simulink model "adapt_visodo05_RC"  (Simulink 7.5)
settings: Solver=FixedStepDiscrete  StartTime=0.0  StopTime=100  FixedStep=1  RelTol=1e-3
undefined symbols (not defined in the file): L, R
libraries: simulink x2, vipmorphops x1, vipsnks x1
(part 1 of 2)
CloseFcn:
  | rtwprivate ssgencode ModelCloseRequest adapt_visodo05_batch_adapt
settings Model: Creator=jfabia02  LastModifiedBy=jfabia02  SimulationMode=external  ExtModeEnableFloating=off  ExtModeArchiveFileName=model_output  ExtModeArchiveDirName=C:\RTtools\VU-RLNX\RLNX\RLNX\Simulink Models
settings DataIOCC: ExternalInput=[t,u]
settings DebuggingCC: UnderspecifiedInitializationDetection=Simplified  UnconnectedInputMsg=none  UnconnectedOutputMsg=none  UnconnectedLineMsg=none
settings RTWCC: SystemTargetFile=rlnx.tlc  GenCodeOnly=on  TemplateMakefile=rlnx_ubuntu.tmf  Description=Linux Real-Time Target  GenerateReport=on  ProcessScript=rlnx_make_rtw_hook  LaunchReport=on
settings CodeAppCC: GenerateComments=off  SimulinkBlockComments=off
settings STFCustomTargetCC: TargetFunctionLibrary=GNU99 (GNU)  ModelReferenceCompliant=off  GeneratePreprocessorConditionals=Disable all  MatFileLogging=on  SystemTargetFile=rlnx.tlc
settings GRTTargetCC: TargetFunctionLibrary=GNU99 (GNU)  ModelReferenceCompliant=off  ParMdlRefBuildCompliant=off  CompOptLevelCompliant=off  ExtMode=on  ExtModeMexArgs='10.0.0.2'
settings CustomProperty: DataType=string  Value=-lm -ldl /matlab_includes/libfreenect/build/lib/libfreenect.so.0.0.1
settings EnumStrPairs: String=PC

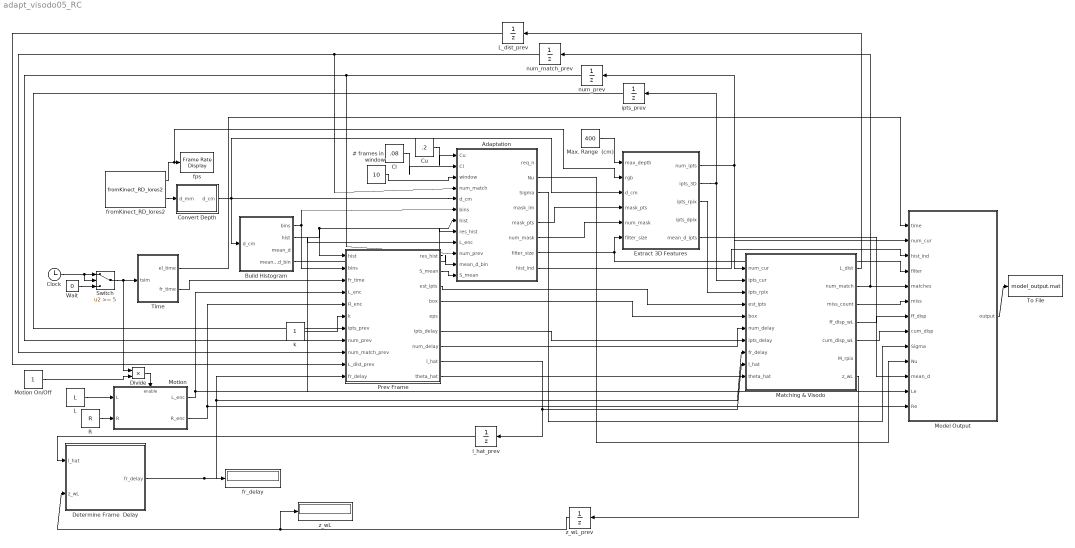
== system adapt_visodo05_RC ==
  # frames in  window : Constant  Value=10  OutDataType=fixdt(1, 16)  OutScaling=2^0
  Adaptation : Subsystem
  Build Histogram : Stateflow chart  TreatAsAtomicUnit=on
  Cl : Constant  Value=.08  OutDataType=fixdt(1, 16)  OutScaling=2^0
  Clock : Clock
      settings: Decimation=10
  Convert Depth : Subsystem
  Cu : Constant  Value=.2  OutDataType=fixdt(1, 16)  OutScaling=2^0
  Determine Frame  Delay : Stateflow chart  TreatAsAtomicUnit=on
  Divide : Product  Inputs=**  OutDataType=fixdt(1, 16)  OutScaling=2^-10
  Extract 3D Features : Subsystem
  L : Constant  Value=L  OutDataType=fixdt(1, 16)  OutScaling=2^0
  L_dist_prev : UnitDelay  X0=zeros(2,1000)  SampleTime=-1
  Matching & Visodo : Subsystem
  Max. Range  (cm) : Constant  Value=400  OutDataType=fixdt(1, 16)  OutScaling=2^0
  Model Output : Stateflow chart  TreatAsAtomicUnit=on
  Motion : Subsystem
  Motion On/Off : Constant  OutDataType=fixdt(1, 16)  OutScaling=2^0
  Prev Frame : Subsystem
  R : Constant  Value=R  OutDataType=fixdt(1, 16)  OutScaling=2^0
  Switch : Switch  Threshold=5  OutDataType=fixdt(1, 16)  OutScaling=2^0
  Time : Subsystem
  To File : ToFile  Filename=model_output.mat  MatrixName=output
  Wait : Constant  Value=0  OutDataType=fixdt(1, 16)  OutScaling=2^0
  fps : vipsnks/Frame Rate Display  DialogController=vipDDGCreate  DialogControllerArgs=DataTag0  UpdateRate=10
  fr_delay : Display
  fromKinect_RD_lores2 : S-Function  FunctionName=fromKinect_RD_lores2  EnableBusSupport=off
      mask Display: image(imread('C:\RTtools\VU-RLNX\RLNX\RLNX\Simulink Models\kinectimage.jpeg'))
  ipts_prev : UnitDelay  SampleTime=-1
  k : Constant  OutDataType=fixdt(1, 16)  OutScaling=2^0
  l_hat_prev : UnitDelay  SampleTime=-1
  num_match_prev : UnitDelay  SampleTime=-1
  num_prev : UnitDelay  SampleTime=-1
  z_wL : Display
  z_wL_prev : UnitDelay  SampleTime=-1
  wires:
  Max. Range  (cm)/1 -> Extract 3D Features/1(max_depth)
  Convert Depth/1(d_cm) -> Extract 3D Features/3(d_cm), Build Histogram/1(d_cm), Adaptation/5(d_cm)
  ipts_prev/1 -> Prev Frame/7(ipts_prev)
  num_prev/1 -> Prev Frame/8(num_prev), Adaptation/10(num_prev)
  k/1 -> Prev Frame/6(k)
  Build Histogram/2(hist) -> Prev Frame/1(hist), Adaptation/7(hist)
  # frames in  window/1 -> Adaptation/3(window)
  Matching & Visodo/2(num_match) -> num_match_prev/1, Model Output/5(matches)
  num_match_prev/1 -> Prev Frame/9(num_match_prev), Adaptation/4(num_match)
  Prev Frame/3(est_ipts) -> Matching & Visodo/4(est_ipts)
  Prev Frame/4(box) -> Matching & Visodo/5(box)
  Extract 3D Features/3(ipts_rpix) -> Matching & Visodo/3(ipts_rpix)
  Extract 3D Features/2(ipts_3D) -> Matching & Visodo/2(ipts_cur), ipts_prev/1
  Prev Frame/1(res_hist) -> Adaptation/8(res_hist)
  Adaptation/7(filter_size) -> Extract 3D Features/6(filter_size), Model Output/4(filter)
  Build Histogram/1(bins) -> Prev Frame/2(bins), Adaptation/6(bins)
  Matching & Visodo/1(" L_dist") -> L_dist_prev/1
  L_dist_prev/1 -> Prev Frame/10(L_dist_prev)
  Adaptation/5(mask_pts) -> Extract 3D Features/4(mask_pts)
  Adaptation/6(num_mask) -> Extract 3D Features/5(num_mask)
  Extract 3D Features/1(num_ipts) -> Matching & Visodo/1(num_cur), num_prev/1, Model Output/2(num_cur)
  Prev Frame/7(num_delay) -> Matching & Visodo/6(num_delay)
  Prev Frame/6(ipts_delay) -> Matching & Visodo/7(ipts_delay)
  Cu/1 -> Adaptation/1(Cu)
  Cl/1 -> Adaptation/2(Cl)
  Prev Frame/8(l_hat) -> Matching & Visodo/9(l_hat), l_hat_prev/1
  Prev Frame/9(theta_hat) -> Matching & Visodo/10(theta_hat)
  Build Histogram/4(mean_d_bin) -> Adaptation/11(mean_d_bin)
  Determine Frame  Delay/1(fr_delay) -> fr_delay/1, Prev Frame/11(fr_delay), Matching & Visodo/8(fr_delay)
  z_wL_prev/1 -> Determine Frame  Delay/2(z_wL), z_wL/1
  l_hat_prev/1 -> Determine Frame  Delay/1(l_hat)
  Matching & Visodo/7(z_wL) -> z_wL_prev/1
  Prev Frame/2(S_mean) -> Adaptation/12(S_mean)
  Clock/1 -> Switch/2, Switch/1
  Switch/1 -> Time/1(tsim), Divide/1
  Wait/1 -> Switch/3
  Motion On/Off/1 -> Divide/2
  L/1 -> Motion/1(L)
  R/1 -> Motion/2(R)
  Divide/1 -> Motion/Enable
  fromKinect_RD_lores2/2 -> Convert Depth/1(d_mm)
  fromKinect_RD_lores2/1 -> Extract 3D Features/2(rgb), fps/1
  Time/2(fr_time) -> Prev Frame/3(fr_time)
  Model Output/1(output) -> To File/1
  Time/1(el_time) -> Model Output/1(time)
  Adaptation/8(hist_ind) -> Model Output/3(hist_ind)
  Matching & Visodo/3(miss_count) -> Model Output/6(miss)
  Matching & Visodo/4(ff_disp_wL) -> Model Output/7(ff_disp)
  Matching & Visodo/5(cum_disp_wL) -> Model Output/8(cum_disp)
  Adaptation/2(Nu) -> Model Output/10(Nu)
  Adaptation/3(Sigma) -> Model Output/9(Sigma)
  Extract 3D Features/5(mean_d_ipts) -> Model Output/11(mean_d)
  Motion/1(L_enc) -> Prev Frame/4(L_enc), Adaptation/9(L_enc), Model Output/12(Le)
  Motion/2(R_enc) -> Prev Frame/5(R_enc), Model Output/13(Re)

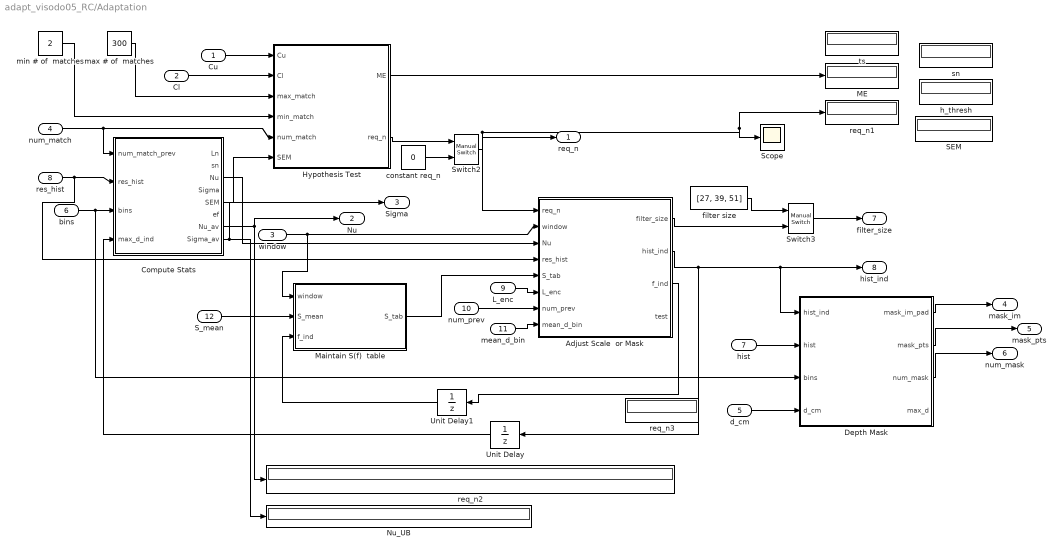
== system adapt_visodo05_RC/Adaptation ==
  Cu : Inport
  Cl : Inport  Port=2
  window : Inport  Port=3
  num_match : Inport  Port=4
  d_cm : Inport  Port=5
  bins : Inport  Port=6
  hist : Inport  Port=7  OutDataType=fixdt(1, 16)  OutScaling=2^0
  res_hist : Inport  Port=8
  L_enc : Inport  Port=9  OutDataType=fixdt(1, 16)  OutScaling=2^0
  num_prev : Inport  Port=10  OutDataType=fixdt(1, 16)  OutScaling=2^0
  mean_d_bin : Inport  Port=11  OutDataType=fixdt(1, 16)  OutScaling=2^0
  S_mean : Inport  Port=12
  Adjust Scale  or Mask : Stateflow chart  TreatAsAtomicUnit=on
  Compute Stats : Stateflow chart  TreatAsAtomicUnit=on
  Depth Mask : Stateflow chart  TreatAsAtomicUnit=on
  Hypothesis Test : Stateflow chart  TreatAsAtomicUnit=on
  ME : Display
  Maintain S(f)  table : Stateflow chart  TreatAsAtomicUnit=on
  Nu_UB : Display
  SEM : Display
  Scope : Scope
      settings: TimeRange=1000  YMin=-2  YMax=2
  Switch2 : simulink/Signal Routing/Manual Switch  SystemSampleTime=-1  sw=1  action=0  varsize=off
  Switch3 : simulink/Signal Routing/Manual Switch  SystemSampleTime=-1  sw=0  action=0  varsize=off
  Unit Delay : UnitDelay  X0=2  SampleTime=-1
  Unit Delay1 : UnitDelay  X0=2  SampleTime=-1
  constant req_n : Constant  Value=0  OutDataType=fixdt(1, 16)  OutScaling=2^0
  filter size : Constant  Value=[27, 39, 51]  VectorParams1D=off  OutDataType=fixdt(1, 16)  OutScaling=2^0
  h_thresh : Display
  max # of  matches : Constant  Value=300  OutDataType=fixdt(1, 16)  OutScaling=2^0
  min # of  matches : Constant  Value=2  OutDataType=fixdt(1, 16)  OutScaling=2^0
  req_n1 : Display
  req_n2 : Display
  req_n3 : Display
  sn : Display
  ts : Display
  req_n : Outport
  Nu : Outport  Port=2
  Sigma : Outport  Port=3
  mask_im : Outport  Port=4
  mask_pts : Outport  Port=5
  num_mask : Outport  Port=6
  filter_size : Outport  Port=7
  hist_ind : Outport  Port=8
  wires:
  Hypothesis Test/1(ME) -> ME/1
  num_match/1 -> Hypothesis Test/5(num_match), Compute Stats/1(num_match_prev)
  window/1 -> Adjust Scale  or Mask/2(window), Maintain S(f)  table/1(window)
  res_hist/1 -> Compute Stats/2(res_hist), Adjust Scale  or Mask/4(res_hist)
  bins/1 -> Compute Stats/3(bins), Depth Mask/3(bins)
  Compute Stats/3(Nu) -> Adjust Scale  or Mask/3(Nu)
  d_cm/1 -> Depth Mask/4(d_cm)
  Depth Mask/3(num_mask) -> num_mask/1
  Depth Mask/1(mask_im_pad) -> mask_im/1
  Depth Mask/2(mask_pts) -> mask_pts/1
  hist/1 -> Depth Mask/2(hist)
  Adjust Scale  or Mask/2(hist_ind) -> Unit Delay/1, hist_ind/1, Depth Mask/1(hist_ind)
  Hypothesis Test/2(req_n) -> Switch2/1
  Switch2/1 -> Adjust Scale  or Mask/1(req_n), req_n/1, Scope/1, req_n1/1
  constant req_n/1 -> Switch2/2
  Adjust Scale  or Mask/1(filter_size) -> Switch3/2
  Switch3/1 -> filter_size/1
  filter size/1 -> Switch3/1
  min # of  matches/1 -> Hypothesis Test/4(min_match)
  L_enc/1 -> Adjust Scale  or Mask/6(L_enc)
  Unit Delay/1 -> Compute Stats/4(max_d_ind)
  Compute Stats/5(SEM) -> Hypothesis Test/6(SEM)
  Cu/1 -> Hypothesis Test/1(Cu)
  num_prev/1 -> Adjust Scale  or Mask/7(num_prev)
  mean_d_bin/1 -> Adjust Scale  or Mask/8(mean_d_bin)
  Cl/1 -> Hypothesis Test/2(Cl)
  max # of  matches/1 -> Hypothesis Test/3(max_match)
  Adjust Scale  or Mask/3(f_ind) -> Unit Delay1/1
  Unit Delay1/1 -> Maintain S(f)  table/3(f_ind)
  S_mean/1 -> Maintain S(f)  table/2(S_mean)
  Maintain S(f)  table/1(S_tab) -> Adjust Scale  or Mask/5(S_tab)
  Compute Stats/7(Nu_av) -> req_n2/1, Nu/1
  Compute Stats/8(Sigma_av) -> Nu_UB/1, Sigma/1

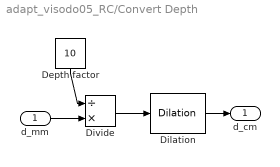
== system adapt_visodo05_RC/Convert Depth ==
  d_mm : Inport
  Depth factor : Constant  Value=10  OutDataType=fixdt(1, 16)  OutScaling=2^0
  Dilation : vipmorphops/Dilation  nhoodsrc=Specify via dialog  strel=[2 2; 2 2]
  Divide : Product  Inputs=/*  OutDataType=fixdt(1, 16)  OutScaling=2^-10
  d_cm : Outport
  wires:
  Divide/1 -> Dilation/1
  Depth factor/1 -> Divide/1
  d_mm/1 -> Divide/2
  Dilation/1 -> d_cm/1

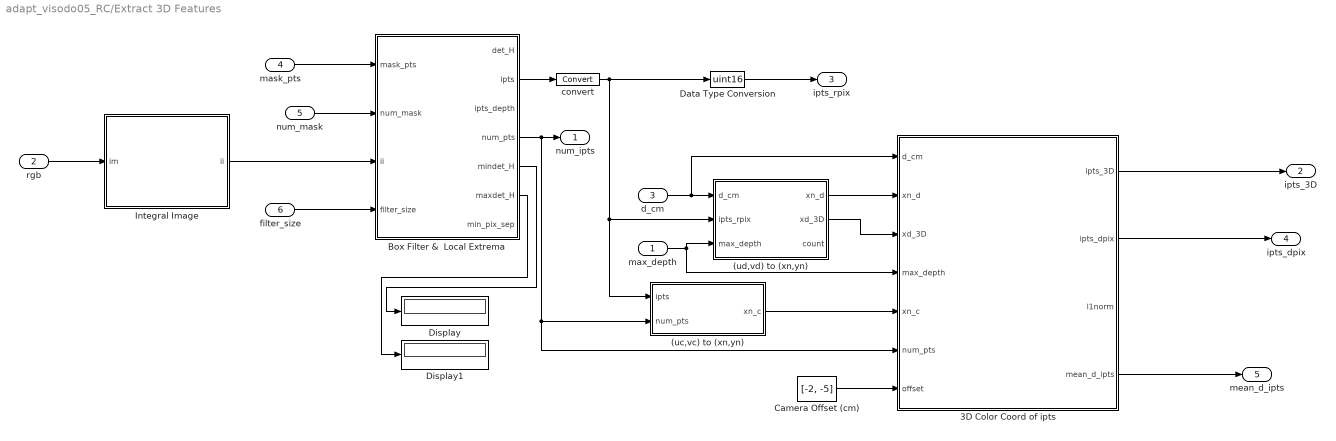
== system adapt_visodo05_RC/Extract 3D Features ==
  max_depth : Inport  OutDataType=fixdt(1, 16)  OutScaling=2^0
  rgb : Inport  Port=2
  d_cm : Inport  Port=3
  mask_pts : Inport  Port=4
  num_mask : Inport  Port=5
  filter_size : Inport  Port=6  OutDataType=fixdt(1, 16)  OutScaling=2^0
  (uc,vc) to (xn,yn) : Stateflow chart  TreatAsAtomicUnit=on
  (ud,vd) to (xn,yn) : Stateflow chart  TreatAsAtomicUnit=on
  3D Color Coord of ipts : Stateflow chart  TreatAsAtomicUnit=on
  Box Filter &  Local Extrema : Stateflow chart  TreatAsAtomicUnit=on
  Camera Offset (cm) : Constant  Value=[-2, -5]  OutDataTypeMode=double  OutDataType=fixdt(1, 16)  OutScaling=2^0  OutDataTypeStr=double
  Data Type Conversion : DataTypeConversion  OutDataTypeMode=uint16  OutDataType=fixdt(1, 16)  OutScaling=2^0  OutDataTypeStr=uint16
  Display : Display
  Display1 : Display
  Integral Image : Stateflow chart  TreatAsAtomicUnit=on
  convert : DataTypeConversion  OutDataType=fixdt(1, 16)  OutScaling=2^0
  num_ipts : Outport
  ipts_3D : Outport  Port=2
  ipts_rpix : Outport  Port=3
  ipts_dpix : Outport  Port=4
  mean_d_ipts : Outport  Port=5
  wires:
  rgb/1 -> Integral Image/1(im)
  filter_size/1 -> Box Filter &  Local Extrema/4(filter_size)
  Box Filter &  Local Extrema/2(ipts) -> convert/1
  Data Type Conversion/1 -> ipts_rpix/1
  Box Filter &  Local Extrema/4(num_pts) -> num_ipts/1, (uc,vc) to (xn,yn)/2(num_pts), 3D Color Coord of ipts/6(num_pts)
  Integral Image/1(ii) -> Box Filter &  Local Extrema/3(ii)
  mask_pts/1 -> Box Filter &  Local Extrema/1(mask_pts)
  num_mask/1 -> Box Filter &  Local Extrema/2(num_mask)
  (ud,vd) to (xn,yn)/1(xn_d) -> 3D Color Coord of ipts/2(xn_d)
  (ud,vd) to (xn,yn)/2(xd_3D) -> 3D Color Coord of ipts/3(xd_3D)
  (uc,vc) to (xn,yn)/1(xn_c) -> 3D Color Coord of ipts/5(xn_c)
  d_cm/1 -> (ud,vd) to (xn,yn)/1(d_cm), 3D Color Coord of ipts/1(d_cm)
  Camera Offset (cm)/1 -> 3D Color Coord of ipts/7(offset)
  max_depth/1 -> (ud,vd) to (xn,yn)/3(max_depth), 3D Color Coord of ipts/4(max_depth)
  3D Color Coord of ipts/1(ipts_3D) -> ipts_3D/1
  convert/1 -> Data Type Conversion/1, (ud,vd) to (xn,yn)/2(ipts_rpix), (uc,vc) to (xn,yn)/1(ipts)
  Box Filter &  Local Extrema/5(mindet_H) -> Display/1
  Box Filter &  Local Extrema/6(maxdet_H) -> Display1/1
  3D Color Coord of ipts/2(ipts_dpix) -> ipts_dpix/1
  3D Color Coord of ipts/4(mean_d_ipts) -> mean_d_ipts/1

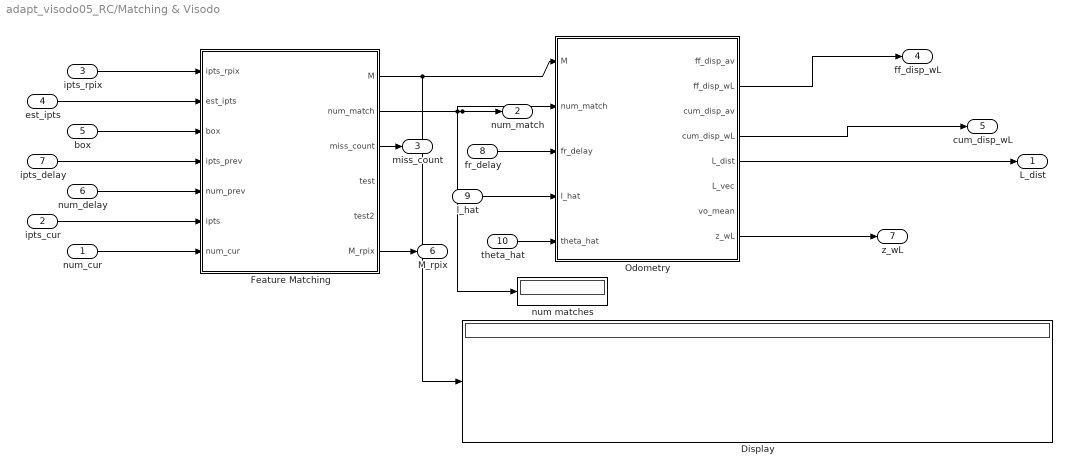
== system adapt_visodo05_RC/Matching & Visodo ==
  num_cur : Inport
  ipts_cur : Inport  Port=2
  ipts_rpix : Inport  Port=3  OutDataType=fixdt(1, 16)  OutScaling=2^0
  est_ipts : Inport  Port=4
  box : Inport  Port=5
  num_delay : Inport  Port=6
  ipts_delay : Inport  Port=7
  fr_delay : Inport  Port=8
  l_hat : Inport  Port=9
  theta_hat : Inport  Port=10
  Display : Display
  Feature Matching : Stateflow chart  TreatAsAtomicUnit=on
  Odometry : Stateflow chart  TreatAsAtomicUnit=on
  num matches : Display
  " L_dist" : Outport
  num_match : Outport  Port=2
  miss_count : Outport  Port=3
  ff_disp_wL : Outport  Port=4
  cum_disp_wL : Outport  Port=5
  M_rpix : Outport  Port=6  PortDimensions=[2 1000]
  z_wL : Outport  Port=7
  wires:
  Feature Matching/3(miss_count) -> miss_count/1
  Feature Matching/1(M) -> Odometry/1(M), Display/1
  Feature Matching/2(num_match) -> num_match/1, Odometry/2(num_match), num matches/1
  ipts_rpix/1 -> Feature Matching/1(ipts_rpix)
  ipts_cur/1 -> Feature Matching/6(ipts)
  num_cur/1 -> Feature Matching/7(num_cur)
  ipts_delay/1 -> Feature Matching/4(ipts_prev)
  num_delay/1 -> Feature Matching/5(num_prev)
  est_ipts/1 -> Feature Matching/2(est_ipts)
  box/1 -> Feature Matching/3(box)
  Odometry/5(L_dist) -> " L_dist"/1
  Feature Matching/6(M_rpix) -> M_rpix/1
  Odometry/2(ff_disp_wL) -> ff_disp_wL/1
  Odometry/4(cum_disp_wL) -> cum_disp_wL/1
  fr_delay/1 -> Odometry/3(fr_delay)
  l_hat/1 -> Odometry/4(l_hat)
  theta_hat/1 -> Odometry/5(theta_hat)
  Odometry/8(z_wL) -> z_wL/1

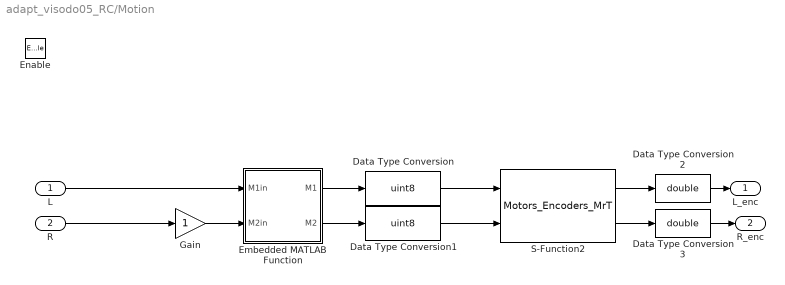
== system adapt_visodo05_RC/Motion ==
  L : Inport  OutDataType=fixdt(1, 16)  OutScaling=2^0
  R : Inport  Port=2  OutDataType=fixdt(1, 16)  OutScaling=2^0
  Enable : EnablePort
  Data Type Conversion : DataTypeConversion  OutDataTypeMode=uint8  OutDataType=fixdt(1, 16)  OutScaling=2^0  OutDataTypeStr=uint8
  Data Type Conversion1 : DataTypeConversion  OutDataTypeMode=uint8  OutDataType=fixdt(1, 16)  OutScaling=2^0  OutDataTypeStr=uint8
  Data Type Conversion2 : DataTypeConversion  OutDataTypeMode=double  OutDataType=fixdt(1, 16)  OutScaling=2^0  OutDataTypeStr=double
  Data Type Conversion3 : DataTypeConversion  OutDataTypeMode=double  OutDataType=fixdt(1, 16)  OutScaling=2^0  OutDataTypeStr=double
  Embedded MATLAB Function : Stateflow chart  TreatAsAtomicUnit=on
  Gain : Gain  ParameterDataType=fixdt(1, 16)  ParameterScaling=2^0  OutDataType=fixdt(1, 16)  OutScaling=2^0
  S-Function2 : S-Function  FunctionName=Motors_Encoders_MrT  EnableBusSupport=off
  L_enc : Outport  InitialOutput=0
  R_enc : Outport  Port=2  InitialOutput=0
  wires:
  L/1 -> Embedded MATLAB Function/1(M1in)
  Gain/1 -> Embedded MATLAB Function/2(M2in)
  Data Type Conversion1/1 -> S-Function2/2
  Data Type Conversion/1 -> S-Function2/1
  Embedded MATLAB Function/2(M2) -> Data Type Conversion1/1
  Embedded MATLAB Function/1(M1) -> Data Type Conversion/1
  S-Function2/1 -> Data Type Conversion2/1
  S-Function2/2 -> Data Type Conversion3/1
  R/1 -> Gain/1
  Data Type Conversion2/1 -> L_enc/1
  Data Type Conversion3/1 -> R_enc/1

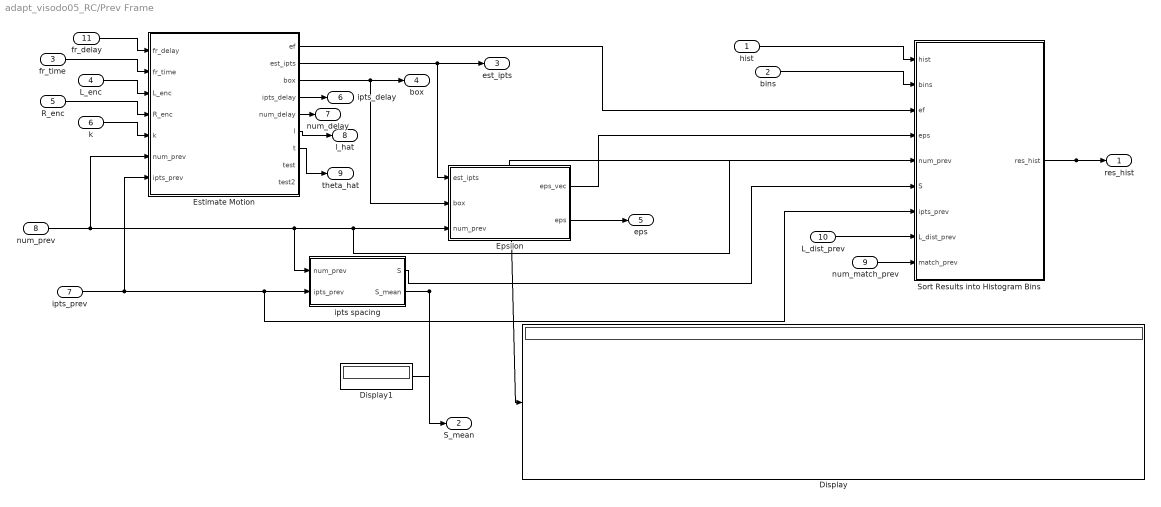
== system adapt_visodo05_RC/Prev Frame ==
  hist : Inport
  bins : Inport  Port=2
  fr_time : Inport  Port=3
  L_enc : Inport  Port=4
  R_enc : Inport  Port=5
  k : Inport  Port=6
  ipts_prev : Inport  Port=7
  num_prev : Inport  Port=8
  num_match_prev : Inport  Port=9
  L_dist_prev : Inport  Port=10
  fr_delay : Inport  Port=11
  Display : Display
  Display1 : Display
  Epsilon : Stateflow chart  TreatAsAtomicUnit=on
  Estimate Motion : Stateflow chart  TreatAsAtomicUnit=on
  Sort Results into Histogram Bins : Stateflow chart  TreatAsAtomicUnit=on
  ipts spacing : Stateflow chart  TreatAsAtomicUnit=on
  res_hist : Outport
  S_mean : Outport  Port=2
  est_ipts : Outport  Port=3
  box : Outport  Port=4
  eps : Outport  Port=5
  ipts_delay : Outport  Port=6
  num_delay : Outport  Port=7
  l_hat : Outport  Port=8
  theta_hat : Outport  Port=9
  wires:
  Estimate Motion/2(est_ipts) -> est_ipts/1, Epsilon/1(est_ipts)
  Sort Results into Histogram Bins/1(res_hist) -> res_hist/1, Display/1
  num_prev/1 -> ipts spacing/1(num_prev), Epsilon/3(num_prev), Sort Results into Histogram Bins/5(num_prev), Estimate Motion/6(num_prev)
  ipts_prev/1 -> ipts spacing/2(ipts_prev), Sort Results into Histogram Bins/7(ipts_prev), Estimate Motion/7(ipts_prev)
  hist/1 -> Sort Results into Histogram Bins/1(hist)
  Estimate Motion/1(ef) -> Sort Results into Histogram Bins/3(ef)
  ipts spacing/1(S) -> Sort Results into Histogram Bins/6(S)
  Epsilon/1(eps_vec) -> Sort Results into Histogram Bins/4(eps)
  bins/1 -> Sort Results into Histogram Bins/2(bins)
  L_dist_prev/1 -> Sort Results into Histogram Bins/8(L_dist_prev)
  num_match_prev/1 -> Sort Results into Histogram Bins/9(match_prev)
  Estimate Motion/5(num_delay) -> num_delay/1
  fr_delay/1 -> Estimate Motion/1(fr_delay)
  fr_time/1 -> Estimate Motion/2(fr_time)
  L_enc/1 -> Estimate Motion/3(L_enc)
  R_enc/1 -> Estimate Motion/4(R_enc)
  k/1 -> Estimate Motion/5(k)
  Estimate Motion/3(box) -> box/1, Epsilon/2(box)
  Estimate Motion/4(ipts_delay) -> ipts_delay/1
  Epsilon/2(eps) -> eps/1
  Estimate Motion/6(l) -> l_hat/1
  Estimate Motion/7(t) -> theta_hat/1
  ipts spacing/2(S_mean) -> Display1/1, S_mean/1

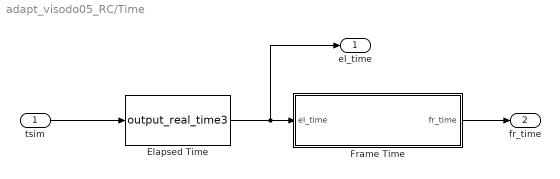
== system adapt_visodo05_RC/Time ==
  tsim : Inport  OutDataType=fixdt(1, 16)  OutScaling=2^0
  Elapsed Time : S-Function  FunctionName=output_real_time3  EnableBusSupport=off
  Frame Time : Stateflow chart  TreatAsAtomicUnit=on
  el_time : Outport
  fr_time : Outport  Port=2
  wires:
  tsim/1 -> Elapsed Time/1
  Elapsed Time/1 -> Frame Time/1(el_time), el_time/1
  Frame Time/1(fr_time) -> fr_time/1

== matlab function Build Histogram ==
  data: bins output double; d_cm input double; hist output double; mean_d output double; mean_d_bin output double
function [bins,hist, mean_d, mean_d_bin] = hist(d_cm)
% function builds histogram with non-uniform bins

% Q=1.4e-5*z^2
% 1.4e-5(z2^2 - z1^2) = C  %% constant change in Q over each bin
% if first bin is 50-125cm...
% C=0.18375  ===>  z2 = sqrt(13125+z1^2);

persistent z_pers
if isempty(z_pers)
    z_pers=zeros(2,19);
    z_pers(:,1)=[50; 125];
    for i=2:19
        z_pers(1,i)=z_pers(2,i-1); % front of bin
        z_pers(2,i)=sqrt(13125+z_pers(1,i)^2); % back of bin
    end
end
z=z_pers;

h=size(d_cm,1);
w=size(d_cm,2);
hist=zeros(1,19);
bins=zeros(2,19);
hist_pix=0;
sum_d=0;

for i=1:w
    for j=1:h
        n=1;
        if d_cm(j,i)<50 || d_cm(j,i)>500
            break
        else
            hist_pix=hist_pix+1; % counter of pixels in histogram
            sum_d=sum_d+d_cm(j,i); % running sum of depth of pixels in histogram
            for n=1:19
                z2=z(2,n);
                if d_cm(j,i)<=z2
                    hist(1,n)=hist(1,n)+1;
                    break
                end
            end
        end
    end
end
% calculate average depth of pixels in histogram and find associated bin
mean_d=sum_d/hist_pix;
mean_d_bin=1;
for n=1:19
    z2=z(2,n);
    if mean_d<=z2
        mean_d_bin=n;
        break
    end
end
bins(1:2,:)=z;

== matlab function Determine Frame Delay ==
  data: l_hat input double; fr_delay output double; z_wL input double
function fr_delay = calc_fr_delay(l_hat, z_wL)
% function calculates necessary frame delay based on weighted mean depth of matches, z_wL,
%   and estimated motion from encoders, l_hat

Qz_wL=1.4e-5*(z_wL)^2; % quantization error in depth sensor at weighted mean depth of matches

if l_hat==0
    fr_delay=0;
else
    fr_delay=ceil(Qz_wL/l_hat)+2;
end

if fr_delay>9
    fr_delay=9;
elseif isnan(fr_delay)
    fr_delay=0;
end

== matlab function Adaptation/Hypothesis Test ==
  data: Cu input double; Cl input double; max_match input double; min_match input double; ME output double; num_match input double; SEM input double; req_n output double
function [ME, req_n] = req_num(Cu,Cl,max_match,min_match,num_match,SEM)
% function determines whether or not there are a sufficient number of ipts
%   req_n=-1 ==> not enough features
%   req_n= 0 ==> number of features is just right
%   req_n= 1 ==> too many features

req_n=0;

persistent t_l
if isempty(t_l) %LUT of t_scores
    t_l=[12.71 4.303 3.182 2.776 2.571 2.447 2.365 2.306 2.262 2.228 2.201 2.179 ...
        2.16 2.145 2.131 2.12 2.11 2.101 2.093 2.086 2.08 2.074 2.069 2.064 2.06 ...
        2.056 2.052 2.048 2.045 2.042]; 
end

n=num_match;
df=n-1;

if n<=30 && n>=min_match
    ta2=t_l(df); % t_alpha/2
elseif n>30
    ta2=1.96;
else
    ta2=0;
end
ME=ta2*SEM; % margin of error

% hypothesis test
if n<min_match
    req_n=-1;
elseif n>max_match
    req_n=1;
else
    if ME>Cu % insufficient matches
        req_n=-1;
    elseif ME<=Cu && ME>=Cl % just right
        req_n=0;
    elseif ME<Cl % too many matches
        req_n=1;
    end
end

== matlab function Extract 3D Features/Integral Image ==
  data: im input double; ii output double
function ii = integral_image(im)
% function input is image, im
% output is integral image, ii
im = double(im);
height = size(im,1);
width = size(im,2);
ii = double(zeros(height, width));
col_sum = zeros(height,1);

ii(1,1) = double(im(1,1));
% first column
for j = 2:height
    ii(j,1) = im(j,1) + ii(j-1,1);
end
% first row
for i = 2:width
    ii(1,i) = im(1,i) + ii(1, i-1);
end
% rest of image
for i = 2:width
    col_sum(1,1) = im(1,i);
    for j = 2:height
        col_sum(j,1) = im(j,i) + col_sum(j-1,1);
        ii(j,i) = col_sum(j,1) + ii(j,i-1);
    end
end

== matlab function Extract 3D Features/Box Filter & Local Extrema ==
  data: mask_pts input double; num_mask input double; det_H output double; ipts output double; ipts_depth output double; ii input double; filter_size input double; num_pts output double; mindet_H output double; maxdet_H output double; min_pix_sep output double

function [det_H, ipts,ipts_depth, num_pts, mindet_H, maxdet_H, min_pix_sep]  = box_filter(mask_pts,num_mask,ii, filter_size)
% input is integral image calculated in 'Integral Image'
% ipts across 3 scales:
%   - either 15, 27, 39 
%   - or 27, 39, 51

%%%%%%%%%%%%%%%%%%%%%%%%%%%%%%%%%%%%%%%%%%%%%%%%%%%%%%%%%%%%%%%%%%%%%%%
pos_thres = 0;  % use this threshold to fire on high-contrast areas
neg_thres = 0; % det_H range is generally not symmetric about zero
max_num_ipts = 1000; %%%%% 
min_sep = 0; %% minimum separation, in pixels, between adjacent ipts
%%%%%%%%%%%%%%%%%%%%%%%%%%%%%%%%%%%%%%%%%%%%%%%%%%%%%%%%%%%%%%%%%%%%%%%


h = size(ii,1);
w = size(ii,2);
ipts = uint16(zeros(2,max_num_ipts));
ipts_depth=zeros(1,max_num_ipts);
num_pts = 0;
count = 0;
mask=mask_pts;
min_pix_sep=777;
det_H = zeros(h,w);
mindet_H = 0;
maxdet_H = 0;
Dyy = zeros(h,w);
Dxx = zeros(h,w);
Dxy = zeros(h,w);

persistent fs_pers mask_pts_pers
if isempty(fs_pers)
    fs_pers=zeros(1,3);
% %     fs_pers=filter_size';
    mask_pts_pers=zeros(2,h*w);
    c=0;
    for y=1:h
        for x=1:w
            c=c+1;
            mask_pts_pers(:,c)=[y;x];
        end
    end
end
fs_bands=zeros(2,3);
fs=[0 0 0];

% if mask is empty (off), use all points
if mask_pts(1,1)==0 && mask_pts(2,1)==0
    mask_pts=mask_pts_pers;
end

if fs_pers(1,1)==filter_size(1,1) % filter size hasn't changed
    fs_bands(1,1:3)=fs_pers(1,1:3);
    bands=1;
else
    fs_bands=[fs_pers;filter_size];
    bands=2;
end

for b=1:bands
    fs=fs_bands(b,:);
    
    det_H = zeros(h,w);
    mindet_H = 0;
    maxdet_H = 0;
    Dyy = zeros(h,w);
    Dxx = zeros(h,w);
    Dxy = zeros(h,w);    

    % calculate related filter dimensions
    fc = round(fs(2)/2);
    area = fs(2)*fs(2);
    fs2d3 = (fs(2)/3);

    fc1 = round(fs(1)/2);
    area1 = fs(1)*fs(1);
    fs1d3 = (fs(1)/3);

    fc3 = round(fs(3)/2);
    area3 = fs(3)*fs(3);
    fs3d3 = (fs(3)/3);

% % for i = fc3+1:(w-fc3)
% %     for j = fc3+1:(h-fc3)
    for m=1:num_mask
        j=mask(1,m);
        i=mask(2,m);
        if j>fc && i>fc && j<h-fc && i<w-fc
            % reference points for computing response from integral image
            % o's are Dyy pts, c's are Dxx pts, q's are Dxy pts.
            oj1 = j - fc;
            oi1 = i - (fs2d3); oi2 = oi1; oi3 = oi1; oi4 = oi1;
            oj2 = j - fc + (fs2d3);        
            oj3 = j + fc - (fs2d3)-1;        
            oj4 = j + fc - 1;        
            oj5 = oj1; oj6 = oj2; oj7 = oj3; oj8 = oj4;
            oi5 = i + (fs2d3) -1; oi6 = oi5; oi7 = oi5; oi8 = oi5;
            Dyy(j,i) = 2*(ii(oj7,oi7) - ii(oj6,oi6) -ii(oj3,oi3) + ii(oj2,oi2))...
                       - (ii(oj6,oi6) - ii(oj5,oi5) - ii(oj2,oi2) + ii(oj1,oi1))...
                       - (ii(oj8,oi8) - ii(oj7,oi7) - ii(oj4,oi4) + ii(oj3,oi3));

            ci1 = i - fc;
            cj1 = j - (fs2d3); cj2 = cj1; cj3 = cj1; cj4 = cj1;
            ci2 = i - fc + (fs2d3);        
            ci3 = i + fc - (fs2d3)-1;        
            ci4 = i + fc - 1;        
            ci5 = ci1; ci6 = ci2; ci7 = ci3; ci8 = ci4;
            cj5 = j + (fs2d3) -1; cj6 = cj5; cj7 = cj5; cj8 = cj5;
            Dxx(j,i) = 2*(ii(cj7,ci7) - ii(cj6,ci6) -ii(cj3,ci3) + ii(cj2,ci2))...
                       - (ii(cj6,ci6) - ii(cj5,ci5) - ii(cj2,ci2) + ii(cj1,ci1))...
                       - (ii(cj8,ci8) - ii(cj7,ci7) - ii(cj4,ci4) + ii(cj3,ci3));

            qi1 = i-(fs2d3)-1; qi2 = qi1; qi3 = qi1; qi4=qi1;
            qi5 = i-1; qi6=qi5; qi7=qi5; qi8=qi5;
            qi9 = i; qi10 = i; qi11=i; qi12=i;
            qi13 = i+(fs2d3); qi14=qi13; qi15=qi13; qi16=qi13;
            qj1 = j-(fs2d3)-1; qj5=qj1; qj9=qj1; qj13=qj1;
            qj2 = j-1; qj6=qj2; qj10=qj2; qj14=qj2;
            qj3=j; qj7=j; qj11=j; qj15=j;
            qj4=j+(fs2d3); qj8=qj4; qj12=qj4; qj16=qj4;
            Dxy(j,i) = (ii(qj8,qi8)-ii(qj7,qi7)-ii(qj4,qi4)+ii(qj3,qi3))...
                      + (ii(qj14,qi14)-ii(qj13,qi13)-ii(qj10,qi10)+ii(qj9,qi9))...
                      - (ii(qj6,qi6)-ii(qj5,qi5)-ii(qj2,qi2)+ii(qj1,qi1))...
                      -( ii(qj16,qi16)-ii(qj15,qi15)-ii(qj12,qi12)+ii(qj11,qi11));

            det_H(j,i) = ((Dyy(j,i) * Dxx(j,i)) - (0.81*Dxy(j,i)*Dxy(j,i)))/(area*area);
            if det_H(j,i)>maxdet_H
                maxdet_H = det_H(j,i);
            elseif det_H(j,i)<mindet_H
                mindet_H = det_H(j,i);
            end
        end % if j<....
    % % end % j
    % % end% i
    end %m
    % find local extrema 
    % % for i = fc+1:(w-fc)
    % %     for j = fc+1:(h-fc)
    for m=1:num_mask
        j=mask(1,m);
        i=mask(2,m);
        d=mask(3,m);
        if j>fc3 && i>fc3 && j<h-fc3 && i<w-fc3
            if count < max_num_ipts && i>=fc+3 && j>=fc+3 % && imd(j,i)~=0 && imd(j,i)<max_depth
                p = (det_H(j,i));
                t1 = (det_H(j-1,i-1));
                t2 = (det_H(j,i-1));
                t3 = (det_H(j+1,i-1));
                t4 = (det_H(j-1,i));
                t5 = (det_H(j+1,i));
                t6 = (det_H(j-1,i+1));
                t7 = (det_H(j,i+1));
                t8 = (det_H(j+1,i+1));

                if ((p>pos_thres && p>t1 && p>t2 && p>t3 && p>t4 ...
                   && p>t5 && p>t6 && p>t7 && p>t8) || ...
                   (p<neg_thres && p<t1 && p<t2 && p<t3 && p<t4 ...
                   && p<t5 && p<t6 && p<t7 && p<t8))% && imd(j,i)~=0 && imd(j,i)<max_depth
                    count = count +1;
                    ipts(:,count) = [j;i];
                    ipts_depth(1,count)=d;

                    % delete ipts if too close to previous ipts
                    if count>1 
                        flag=0;

                        for n=1:count-1
                            prox=abs(int16(ipts(1,n))-int16(ipts(1,count))) ...
                               + abs(int16(ipts(2,n))-int16(ipts(2,count)));
                           if prox<=min_sep && flag==0;
                                ipts(:,count) = [0;0]; 
                                ipts_depth(1,count)=0;
                                count =count-1;
                                flag=1; 
                           end
                        end
                    end
    % %             end
                % at this point, have detected ipts in middle band
                % now, need to check against bottom and top bands
                det_H1=0; Dxx1=0; Dyy1=0; Dxy1=0;
                det_H3=0; Dxx3=0; Dyy3=0; Dxy3=0;

                    % build det_H for bottom band, f=1
                    oj1 = j - fc1;
                    oi1 = i - (fs1d3); oi2 = oi1; oi3 = oi1; oi4 = oi1;
                    oj2 = j - fc1 + (fs1d3);        
                    oj3 = j + fc1 - (fs1d3)-1;        
                    oj4 = j + fc1 - 1;        
                    oj5 = oj1; oj6 = oj2; oj7 = oj3; oj8 = oj4;
                    oi5 = i + (fs1d3) -1; oi6 = oi5; oi7 = oi5; oi8 = oi5;
                    Dyy1 = 2*(ii(oj7,oi7) - ii(oj6,oi6) -ii(oj3,oi3) + ii(oj2,oi2))...
                               - (ii(oj6,oi6) - ii(oj5,oi5) - ii(oj2,oi2) + ii(oj1,oi1))...
                               - (ii(oj8,oi8) - ii(oj7,oi7) - ii(oj4,oi4) + ii(oj3,oi3));

                    ci1 = i - fc1;
                    cj1 = j - (fs1d3); cj2 = cj1; cj3 = cj1; cj4 = cj1;
                    ci2 = i - fc1 + (fs1d3);        
                    ci3 = i + fc1 - (fs1d3)-1;        
                    ci4 = i + fc1 - 1;        
                    ci5 = ci1; ci6 = ci2; ci7 = ci3; ci8 = ci4;
                    cj5 = j + (fs1d3) -1; cj6 = cj5; cj7 = cj5; cj8 = cj5;
                    Dxx1 = 2*(ii(cj7,ci7) - ii(cj6,ci6) -ii(cj3,ci3) + ii(cj2,ci2))...
                               - (ii(cj6,ci6) - ii(cj5,ci5) - ii(cj2,ci2) + ii(cj1,ci1))...
                               - (ii(cj8,ci8) - ii(cj7,ci7) - ii(cj4,ci4) + ii(cj3,ci3));

                    qi1 = i-(fs1d3)-1; qi2 = qi1; qi3 = qi1; qi4=qi1;
                    qi5 = i-1; qi6=qi5; qi7=qi5; qi8=qi5;
                    qi9 = i; qi10 = i; qi11=i; qi12=i;
                    qi13 = i+(fs1d3); qi14=qi13; qi15=qi13; qi16=qi13;
                    qj1 = j-(fs1d3)-1; qj5=qj1; qj9=qj1; qj13=qj1;
                    qj2 = j-1; qj6=qj2; qj10=qj2; qj14=qj2;
                    qj3=j; qj7=j; qj11=j; qj15=j;
                    qj4=j+(fs1d3); qj8=qj4; qj12=qj4; qj16=qj4;
                    Dxy1 = (ii(qj8,qi8)-ii(qj7,qi7)-ii(qj4,qi4)+ii(qj3,qi3))...
                              + (ii(qj14,qi14)-ii(qj13,qi13)-ii(qj10,qi10)+ii(qj9,qi9))...
                              - (ii(qj6,qi6)-ii(qj5,qi5)-ii(qj2,qi2)+ii(qj1,qi1))...
                              -( ii(qj16,qi16)-ii(qj15,qi15)-ii(qj12,qi12)+ii(qj11,qi11));

                    det_H1 = ((Dyy1 * Dxx1) - (0.81*Dxy1*Dxy1))/(area1*area1);

                    % build det_H for top band, f=3
                    oj1 = j - fc3;
                    oi1 = i - (fs3d3); oi2 = oi1; oi3 = oi1; oi4 = oi1;
                    oj2 = j - fc3 + (fs3d3);        
                    oj3 = j + fc3 - (fs3d3)-1;        
                    oj4 = j + fc3 - 1;        
                    oj5 = oj1; oj6 = oj2; oj7 = oj3; oj8 = oj4;
                    oi5 = i + (fs3d3) -1; oi6 = oi5; oi7 = oi5; oi8 = oi5;
                    Dyy3 = 2*(ii(oj7,oi7) - ii(oj6,oi6) -ii(oj3,oi3) + ii(oj2,oi2))...
                               - (ii(oj6,oi6) - ii(oj5,oi5) - ii(oj2,oi2) + ii(oj1,oi1))...
                               - (ii(oj8,oi8) - ii(oj7,oi7) - ii(oj4,oi4) + ii(oj3,oi3));

                    ci1 = i - fc3;
                    cj1 = j - (fs3d3); cj2 = cj1; cj3 = cj1; cj4 = cj1;
                    ci2 = i - fc3 + (fs3d3);        
                    ci3 = i + fc3 - (fs3d3)-1;        
                    ci4 = i + fc3 - 1;        
                    ci5 = ci1; ci6 = ci2; ci7 = ci3; ci8 = ci4;
                    cj5 = j + (fs3d3) -1; cj6 = cj5; cj7 = cj5; cj8 = cj5;
                    Dxx3 = 2*(ii(cj7,ci7) - ii(cj6,ci6) -ii(cj3,ci3) + ii(cj2,ci2))...
                               - (ii(cj6,ci6) - ii(cj5,ci5) - ii(cj2,ci2) + ii(cj1,ci1))...
                               - (ii(cj8,ci8) - ii(cj7,ci7) - ii(cj4,ci4) + ii(cj3,ci3));

                    qi1 = i-(fs3d3)-1; qi2 = qi1; qi3 = qi1; qi4=qi1;
                    qi5 = i-1; qi6=qi5; qi7=qi5; qi8=qi5;
                    qi9 = i; qi10 = i; qi11=i; qi12=i;
                    qi13 = i+(fs3d3); qi14=qi13; qi15=qi13; qi16=qi13;
                    qj1 = j-(fs3d3)-1; qj5=qj1; qj9=qj1; qj13=qj1;
                    qj2 = j-1; qj6=qj2; qj10=qj2; qj14=qj2;
                    qj3=j; qj7=j; qj11=j; qj15=j;
                    qj4=j+(fs3d3); qj8=qj4; qj12=qj4; qj16=qj4;
                    Dxy3 = (ii(qj8,qi8)-ii(qj7,qi7)-ii(qj4,qi4)+ii(qj3,qi3))...
                              + (ii(qj14,qi14)-ii(qj13,qi13)-ii(qj10,qi10)+ii(qj9,qi9))...
                              - (ii(qj6,qi6)-ii(qj5,qi5)-ii(qj2,qi2)+ii(qj1,qi1))...
                              -( ii(qj16,qi16)-ii(qj15,qi15)-ii(qj12,qi12)+ii(qj11,qi11));

                    det_H3 = ((Dyy3 * Dxx3) - (0.81*Dxy3*Dxy3))/(area3*area3);

                    % delete if ipts is not max relative to bottom and top bands
                    if (abs(p)>abs(det_H1) && abs(p)>abs(det_H3))
                        continue
                    else
                        ipts(:,count) = [0;0]; 
                        ipts_depth(1,count)=d;
                        count =count-1;      
                    end
                end
            end % if count < max_num_ipts
        end
    % %     end % i        
    % % end % j
    end % m
end %b
% compute minimum separation between adjacent pixels
for c=1:count
    for p=c+1:count
        prox=sqrt((double(ipts(1,p))-double(ipts(1,c)))^2 ...
           + (double(ipts(2,p))-double(ipts(2,c)))^2);
        
       if prox<min_pix_sep
           min_pix_sep=prox;
       end
        
    end
end

fs_pers=filter_size;
num_pts = count; % number of ipts found...could be less than max_num_ipts

== matlab function Adaptation/Maintain S(f) table ==
  data: window input double; S_mean input double; S_tab output double; f_ind input double
function S_tab = S_f_table(window, S_mean, f_ind)
% function maintains and updates table of S as function of filter scale, f

persistent S_tab_pers c_pers S_sum_pers
if isempty(S_tab_pers)
    S_tab_pers=[2 4 7 15 25 40]; % initial table of feature spacing for each scale (from empirical data)
    c_pers=0;
    S_sum_pers=0;
end

S_tab=S_tab_pers;
S_sum=S_sum_pers;;

c=c_pers; % counter inside of window
c=c+1;

if isnan(S_mean) % no features
    S_mean=0;
end

if c<window % inside of window
    S_sum=S_sum+S_mean; % running total of average spacing at current f
else % end of window
    c=0;
    S_win=S_sum/window; % average S inside of window
    S_tab(f_ind)=S_win; 
    S_sum=0;
end



S_tab_pers=S_tab;
c_pers=c;
S_sum_pers=S_sum;

== matlab function Motion/Embedded MATLAB Function ==
  data: M1in input double; M1 output double; M2in input double; M2 output double
function [M1, M2] = MotorPackets(M1in, M2in)
%#eml

M1 = 0;
M2 = 1;

if M1in>2
    M1in = 2;
elseif M1in<0
    M1in = 0;
end
if M2in>2
    M2in = 2;
elseif M2in<0
    M2in = 0;
end

gain = 2/(2^7 - 1);

M1 = M1 + round(M1in/gain)*2;
M2 = M2 + round(M2in/gain)*2;

== matlab function Extract 3D Features/(uc,vc) to (xn,yn) ==
  data: ipts input double; num_pts input double; xn_c output double size=[4 ;1000]
function xn_c  = uc_to_xn(ipts, num_pts)
% function builds LUT for xk and...
% converts ipts in (uc, vc) from 'find local extrema' into (xn, yn)


persistent xk_LUT x_inc y_inc x_init x_fin y_init y_fin uc0 vc0 fxc fyc LUT_x_steps LUT_y_steps
if isempty(xk_LUT)
    %%%% Define grid for xk_LUT %%%%%%%%
    x_inc = .01; % frame rate very sensitive to these values
    y_inc = .02;
    x_init = -0.58;
    x_fin = 0.52;
    y_init = -0.36;
    y_fin = 0.13;
    %%%%%%%%%%%%%%%%%%%%%%%%%%%%%%%%%%%%
    
    
    k1=.1925; k2=-.384; k3=.0022; k4=.0056;
    x = x_init:x_inc:x_fin;
    y = y_init:y_inc:y_fin;

    [xn, yn] = meshgrid(x,y);

    xk=xn.*(1+k1.*(xn.^2+yn.^2)+k2.*(xn.^4+yn.^4+2*xn.^2.*yn.^2)) + 2*k3.*xn.*yn + k4.*(3.*xn.^2+yn.^2);
    yk=yn.*(1+k1.*(xn.^2+yn.^2)+k2.*(xn.^4+yn.^4+2*xn.^2.*yn.^2)) + 2*k4.*xn.*yn + k3.*(3.*yn.^2+xn.^2);

    xk_LUT = zeros(size(xk,1),size(xk,2),2);
    xk_LUT(:,:,1) = xk;
    xk_LUT(:,:,2) = yk;
    
    % rgb intrinsics
    uc0 = 318.2174; vc0 = 262.5753;
    fxc = 531.5340; fyc = 529.7583;
    
    LUT_x_steps = (x_fin-x_init)/x_inc +1;
    LUT_y_steps = (y_fin-y_init)/y_inc +1;
end
max_num_ipts = 1000; %%%%% must be same for 'find_local_extrema', 'uc_to_xk' and 'ipts_to_3Dcolor'
num = max_num_ipts;

xk = zeros(1, num);
yk = zeros(1,num);
xn_c = zeros(4, num);

% convert ipts from (uc, vc) to (xk, yk)
for n = 1:num_pts

    xk(n) = (((2*double(ipts(2,n))) - uc0)/fxc); % image is 1/2 width
    yk(n) = ((2*double(ipts(1,n)+40)) - vc0)/fyc; % image is 1/2 height and cropped at row 40

% use LUT to convert (xk, yk) to (xn, yn)
    metricx = abs(xk_LUT(1,1,1)-xk(n));
    metricy = abs(xk_LUT(1,1,2)-yk(n));
    inx=1; jny=1;
    for i = 1:LUT_x_steps
        for j = 1:LUT_y_steps
            if abs(xk_LUT(j,i,1)-xk(n)) < metricx
                metricx = abs(xk_LUT(j,i,1)-xk(n));
                inx = i; % (xn, yn) indices from xk_LUT
            end
            if abs(xk_LUT(j,i,2)-yk(n)) < metricy
                metricy = abs(xk_LUT(j,i,2)-yk(n));
                jny = j; % (xn, yn) indicies from yk_LUT
            end
        end
    end
    % convert indices to metric
    xnx = x_init + (inx-1)*x_inc;
    yny = y_init + (jny-1)*y_inc;  
    % average values from xk_LUT and yk_LUT
    xn_c(:,n) = [(xnx); (yny); double(ipts(1,n)); double(ipts(2,n))];
      
end

== matlab function Extract 3D Features/(ud,vd) to (xn,yn) ==
  data: d_cm input double; ipts_rpix input double; xn_d output double; xd_3D output double; max_depth input double; count output double
function [xn_d, xd_3D, count]  = d_to_xn(d_cm, ipts_rpix, max_depth)
% function converts all points in depth image into normalized color space (xn,yn)

% define persistent variables
persistent r11 r12 r13 r21 r22 r23 r33 t1 t2 ud0 vd0 fxd fyd
if isempty(r11)
    
    % Rrel from fabian_test_results_good.mat
    r11=0.9999; r12=-0.0071; r13=-0.0078;
    r21=0.0069; r22=0.9997; r23=-0.0240;
    r33= 0.9997; %%r31=0.0080; r32=0.0239;

    % Trel from fabian_test_results_good.mat
    t1=-2.08; t2=0.04; %%t3=0.06;

    % Depth camera intrinsics
    ud0 = 324.1963; vd0 = 232.6185;
    fxd = 590.4609; fyd = 582.7801;
end
%%%%%%%%%%%%%%%%%%%%%%%
max_num_ipts = 1000;

% define ROI to search around each ipts
ROI = 10; % will create search area of (ROI+ROI+1)^2
%%%%%%%%%%%%%%%%%%%%%%%

array_size = (ROI+ROI+1)*(ROI+ROI+1);
xd_3D = zeros(array_size,max_num_ipts,3); % depth signal converted to 3D DEPTH coordinates
xn_d = zeros(array_size,max_num_ipts,2); % depth signal converted to NORMALIZED 3D COLOR coordinates

num_ipts = size(ipts_rpix,2);


count = zeros(1,max_num_ipts);
for n = 1:num_ipts
    % shorten variable names for convenience
    i_j = double(ipts_rpix(1,n));
    i_i = double(ipts_rpix(2,n));
    x=0; y=0; z=0;
    
    if i_i~=0 && i_j~=0
    for i = i_i-ROI:i_i+ROI
        for j = i_j-ROI:i_j+ROI
            count(n) = count(n) +1;
            if d_cm(j,i) <= max_depth && d_cm(j,i) ~=28483 % skip points too far away or out of range (28483)
                
                z = double(d_cm(j,i));
                x = double((z/fxd)*(i*2 - ud0));
                y = double((z/fyd)*((j+40)*2 - vd0));
                xd_3D(count(n),n,1) = x; 
                xd_3D(count(n),n,2) = y; 
                xd_3D(count(n),n,3) = z;

                D = r33*z; % approximation based on relative size of terms in D
                xn_d(count(n),n,1) = (r11*x+r12*y+r13*z+t1)/D;
                xn_d(count(n),n,2) = (r21*x+r22*y+r23*z+t2)/D;

            end
        end
    end
    end
end

== matlab function Extract 3D Features/3D Color Coord of ipts ==
  data: d_cm input double; xn_d input double; xd_3D input double; max_depth input double; xn_c input double size=[4;1000]; num_pts input double; ipts_3D output double; ipts_dpix output double size=[2 1000]; l1norm output double; offset input double; mean_d_ipts output double
function [ipts_3D, ipts_dpix, l1norm, mean_d_ipts]  = ipts_to_3Ddepth(d_cm, xn_d,xd_3D, max_depth, xn_c, num_pts, offset)
% function finds best match between ipts/xn from rgb and xn_d
% and generates 3D_DEPTH coordinates for each ipts


persistent ud0 vd0 fxd fyd
if isempty(ud0)
    % Depth camera intrinsics ('fabian_test_results_good.mat')
    ud0 = 324.1963; vd0 = 232.6185;
    fxd = 590.4609; fyd = 582.7801;
end

max_num_ipts = 1000; %%%%% must be same for 'find_local_extrema', 'uc_to_xk' and 'ipts_to_3Dcolor'
dist_thres = 20; % threshold in pixels for match between ipts_rpix and ipts_dix
ROI = 10;
x_offset=offset(1);
z_offset=offset(2);
  
array_size = (ROI+ROI+1)*(ROI+ROI+1);

ipts_3D = zeros(3,max_num_ipts);
ipts_rpix=uint16(zeros(2,max_num_ipts));
ipts_rpix = uint16(xn_c(3:4,1:max_num_ipts));
ipts_dpix = uint16(zeros(2, max_num_ipts));
l1norm = 1;

% calculate L1norm between each pair of points in xn_d and xn_c
for i = 1:num_pts % loop over all ipts
    % get pix coord of current ipts
    xnx = xn_c(1,i);
    yny = xn_c(2,i);
    i_j = xn_c(3,i);
    i_i = xn_c(4,i);
    
    l1norm = (abs(xn_d(1,i,1)-xnx) + abs(xn_d(1,i,2)-yny));

    for c = 2:array_size
            if (abs(xn_d(c,i,1)-xnx) + abs(xn_d(c,i,2)-yny)) < l1norm 
                l1norm = (abs(xn_d(c,i,1)-xnx) + abs(xn_d(c,i,2)-yny)); 
                ipts_3D(:,i) = [xd_3D(c,i,1)+x_offset; xd_3D(c,i,2); xd_3D(c,i,3)+z_offset]; % adjust for offset of camera
                ipts_dpix(1,i) = uint16((((fyd*ipts_3D(2,i)/ipts_3D(3,i)) + vd0)/2)-40);
                ipts_dpix(2,i) = uint16((fxd*(ipts_3D(1,i)/ipts_3D(3,i)) + ud0)/2);
            end
    end
        
    % zero out bad matches
% %     if (abs(ipts_dpix(1,i)-i_j) + abs(ipts_dpix(2,i)-i_i)) > (dist_thres) ...
% %        || d_cm(ipts_dpix(1,i),ipts_dpix(2,i))>=max_depth
% %         ipts_dpix(:,i) = [0;0];
% %         ipts_rpix(:,i) = [0;0];
% %         ipts_3D(:,i) = [0;0;0];
% %     end
end

mean_d_ipts=mean(ipts_3D(3,1:num_pts));

== matlab function Prev Frame/Estimate Motion ==
  data: fr_delay input double; ef output double; fr_time input double; L_enc input double; R_enc input double; k input double; num_prev input double; ipts_prev input double; est_ipts output double; box output double; ipts_delay output double; num_delay output double; l output double; t output double; test output double; test2 output double
function [ef, est_ipts, box, ipts_delay, num_delay, l,t,test, test2]  = est_mot(fr_delay,fr_time, L_enc, R_enc, k, num_prev,ipts_prev)
% function estimates the current of each previous ipts_3D based on encoder data

max_num_ipts = 1000; %%%%% must be same for 'find_local_extrema', 'uc_to_xk' and 'ipts_to_3Dcolor'
alpha=0.02; % angular uncertainty
delta=.3; % linear uncertainty
ef=zeros(1,1000);
est_ipts = zeros(3,max_num_ipts);
box = zeros(7,max_num_ipts); % contains corners of matching region, [c1x,c1z,c2x,c2z,...].
test=zeros(30,5);
ipts_delay=zeros(3,max_num_ipts); 
test2=zeros(30,5);

persistent prev_ipts10 count10 est_ipts10 ipts_delay10
if isempty(prev_ipts10)
    prev_ipts10=zeros(30,max_num_ipts+1); % matrix to store last 5 ipts + num_ipts, oldest on top
    est_ipts10=zeros(30,max_num_ipts+1);
    ipts_delay10=zeros(30,max_num_ipts);
    count10=0;
end

count10=count10+1;
index=(count10-1)*3+1; % ipts have 3 rows
output_row=count10-fr_delay; % fr_delay=0 uses previous frame (doesn't skip any frames)
output_ind=(output_row-1)*3+1; % ipts have 3 rows
if output_row <=0
    output_row=output_row+10;
    output_ind=(output_row-1)*3+1; % ipts have 3 rows
end


% put current ipts_prev in next row
prev_ipts10(index,1)=num_prev;
prev_ipts10(index:index+2,2:num_prev+1)=ipts_prev(1:3,1:num_prev); % prev_ipts5 gets updated with estimated motion
ipts_delay10(index:index+2,1:num_prev)=ipts_prev(1:3,1:num_prev); % ipts_delay5 only stored prev ipts (doesn't add motion estimate)
% % if num_prev==0
% %     prev_ipts5(index,1)=1;
% %     prev_ipts5(index:index+2,2)=[10;10;10]; % dummy value for case of no ipts
% %     ipts_delay5(index:index+2,2)=[10;10;10]; % dummy value for case of no ipts
% % end

num_delay=prev_ipts10(output_ind,1);
ipts_delay(:,1:num_delay)=ipts_delay10(output_ind:output_ind+2,1:num_delay);
% use est_ipts5 for other 4 rows
for f=1:10
    if f~=count10
        indf=(f-1)*3+1; % ipts have 3 rows
        prev_ipts10(indf:indf+2,:)=est_ipts10(indf:indf+2,:);
    end
end


Vl=L_enc*4.5; % lin. velocity of left wheel
Vr=R_enc*4.5; % lin. vel of right wheel
v=0.5*(Vl+Vr); % lin vel of center of robot
w=(Vr-Vl)/31.5; % ang vel of center of robot (2*half-axle=31.5)

l=v*fr_time;
t=1.5708+w*fr_time;

% estimate current locations for all 10 prev frame ipts
for fr=1:10
    indf=(fr-1)*3+1; % ipts have 3 rows
    num=prev_ipts10(indf,1);
    for i=2:num+1
        rx=0;
        rz=0;
        dh=w*fr_time;
        t1=(dh+pi)/2;
        c12=cos(dh);
        s12=sin(dh);
        s1=sin(t1);
        c1=cos(t1);
        xp=prev_ipts10(indf,i);
        yp=prev_ipts10(indf+1,i);
        zp=prev_ipts10(indf+2,i);
        est_ipts10(indf,1)=num;
        est_ipts10(indf:indf+2,i) = [c12 0 s12;0 1 0; -s12 0 c12]*[xp-l*c1; yp; zp-l*s1]; %% 3DOF forward solution
    end %i
% %     est_ipts5(indf:indf+2,2)
end % f
        
% select row from est_ipts5 for output
num=est_ipts10(output_ind,1);
for i=2:num+1
    xh=est_ipts10(output_ind,i);
    yh=est_ipts10(output_ind+1,i);
    zh=est_ipts10(output_ind+2,i);
    est_ipts(:,i-1)=[xh;yh;zh];

    efx=zh*alpha+l*alpha/2 - delta*(alpha-t-1.5708)/2;
    efz=-xh*alpha-delta+.5*alpha*((t-1.5708)*delta-alpha*(l+delta));
    ef(i-1)=sqrt(efx^2+efz^2);

    sx=abs(k*1.4e-2*xh);
    sy=abs(k*2*2.3e-2*yh);
    sz=abs(k*1.44e-5*zh*zh);

    if xh>=0
        ex_l=k*abs(xh*(cos(-alpha)-1)+zh*sin(-alpha)+l*sin(-alpha));
        ex_r=k*abs(xh*(cos(alpha)-1)+zh*sin(alpha)+l*sin(alpha));

    else
        ex_r=k*abs(xh*(cos(-alpha)-1)+zh*sin(-alpha)+l*sin(-alpha));
        ex_l=k*abs(xh*(cos(alpha)-1)+zh*sin(alpha)+l*sin(alpha));

    end

    left=xh-sx-ex_l;
    right=xh+sx+ex_r;
    top_y=max([yh+sy yh-sy]);
    bot_y=min([yh+sy yh-sy]);
    m=2*xh*sin(alpha)/(left-right);
    ez2=k*(zh*(cos(alpha)-1)-xh*sin(alpha)+l*(cos(alpha)-1)+delta);
    ez4=k*(zh*(cos(alpha)-1)-xh*sin(alpha)+l*(cos(alpha)-1)-delta);
    z2=zh+sz+ez2;
    z4=zh-sz+ez4;

    box(1:7,i-1)=[left;...
                right;...
                m;...
                z2;...
                z4;...
                top_y;...
                bot_y];
end %f

% rest count5 if necessary
if count10==10
    count10=0;
end
 
t=t-1.5708;
test=est_ipts10(:,1:5);
test2=prev_ipts10(:,1:5);

== matlab function Time/Frame Time ==
  data: el_time input double; fr_time output double
function fr_time = frame_time(el_time)
% function computes time between last frame and current frame

persistent prev_time
if isempty(prev_time)
    prev_time = 0;
end

fr_time = el_time-prev_time;

prev_time=el_time;

== matlab function Prev Frame/Sort Results into Histogram Bins ==
  data: hist input double; bins input double; ef input double; eps input double; num_prev input double; S input double; ipts_prev input double; res_hist output double; L_dist_prev input double; match_prev input double
function res_hist = bins(hist, bins, ef, eps, num_prev, S, ipts_prev, L_dist_prev, match_prev)
% function sorts various vectors into histogram bins

iz=zeros(1,1000);
iz(1:num_prev)=ipts_prev(3,1:num_prev); %depth of current features
z2=bins(2,:);
res_hist=zeros(8,19); %[num_ipts; rho; sigma; ef; eps; num_match; L_bins; s_bins]
S_temp=zeros(1000,19); % temporary matrix for sorting sigma values to average
ef_temp=zeros(1000,19);
eps_temp=zeros(1000,19);

for i=1:num_prev
    n=1;
    while n<=19;
        if iz(i)<=z2(n)
                res_hist(1,n)=res_hist(1,n)+1;
                S_temp(res_hist(1,n),n)=S(i);
                ef_temp(res_hist(1,n),n)=ef(i);
                eps_temp(res_hist(1,n),n)=eps(i);
                break
        else
            n=n+1;
        end
    end
end

for n=1:19
    if res_hist(1,n)>0
        res_hist(2,n)=res_hist(1,n)/hist(1,n); % rho
        res_hist(3,n)=median(S_temp(1:res_hist(1,n),n)); %S
        res_hist(4,n)=median(ef_temp(1:res_hist(1,n),n)); %ef
        res_hist(5,n)=median(eps_temp(1:res_hist(1,n),n)); %eps
    end
    % results for matches
    L_temp=zeros(1,1000);
    count=0;
    for m=1:match_prev
        L=L_dist_prev(1,m);
        Lz=L_dist_prev(2,m);
        if n==1 % first bin
            if Lz<=z2(1,n) % if L(m) is in bin n
                count=count+1; %count number matches in nth bin
                L_temp(count)=L; % running total for nth bin
            end
        else
            if Lz<=z2(1,n) && Lz>z2(1,n-1) % if L(m) is in bin n
                count=count+1; %count number matches in nth bin
                L_temp(count)=L; % running total for nth bin     
            end
        end
    end
    res_hist(6,n)=count; % number of matches in bin
    if count~=0
        res_hist(7,n)=mean(L_temp(1:count)); % average L for bin
        res_hist(8,n)=std(L_temp(1:count)); % stddev of L for bin
    end
end
